simulink model "Drone2_simulink1"  (R2024a)
settings: Solver=ode1be  StartTime=0.0  StopTime=inf  RelTol=1e-3
model workspace (MAT data in the model file):
  smiData : object (value not decoded)
settings Model: Creator=admin  LastModifiedBy=admin
settings DataIOCC: SaveOutput=off  SaveTime=off

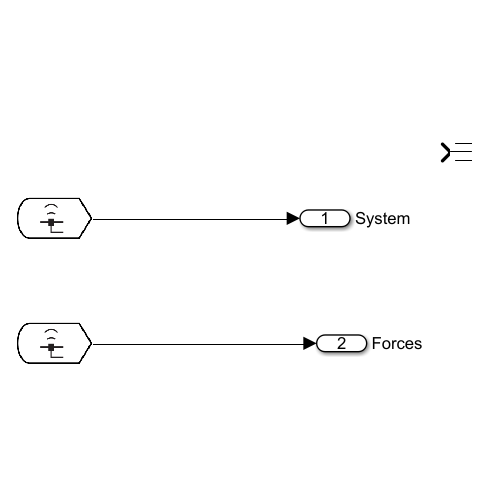
[thumbnail: Simulink's stored preview of the top-level diagram]
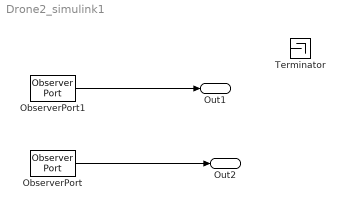
== system Drone2_simulink1 ==
  ObserverPort : ObserverPort
  ObserverPort1 : ObserverPort
  Terminator : Terminator
  Out1 : Outport  SignalName=System
  Out2 : Outport  Port=2  SignalName=Forces
  wires:
  ObserverPort1/1 -> Out1/1
  ObserverPort/1 -> Out2/1
